simulink model "sampleModel2009"  (R2023a)
settings: Solver=VariableStepAuto  StartTime=0.0  StopTime=10.0  RelTol=1e-3
libraries: hdlsllib x4, simulink x3
settings Model: Creator=user1  LastModifiedBy=user1

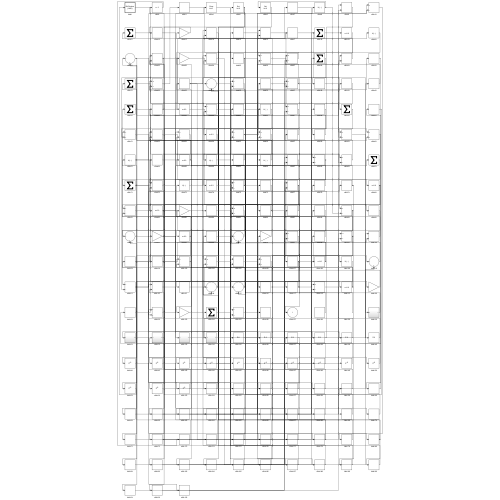
[thumbnail: Simulink's stored preview of the top-level diagram]
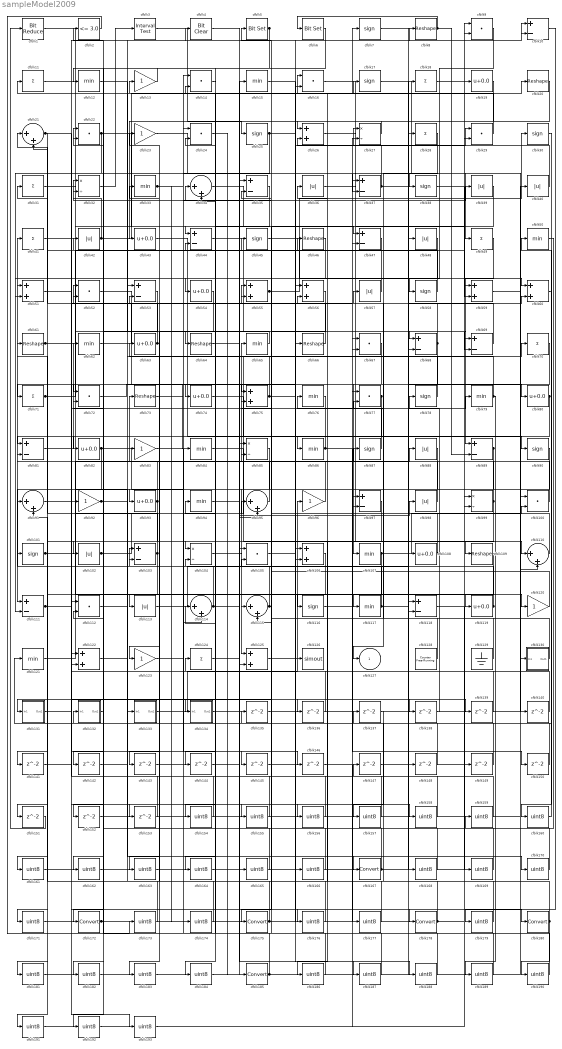
== system sampleModel2009 ==
  cfblk1 : hdlsllib/Logic and Bit Operations/Bit Reduce  mode=AND
  cfblk{10,35,37,44,47,53,68..69,81,89,97,103,111,118} (14 alike) : Sum  Inputs=+-
  cfblk{9,14,16,22,24,29,52,67,72,77,100,105,112} (13 alike) : DotProduct  OutDataTypeStr=Inherit: Inherit via internal rule
  cfblk{7,17,25,30,38,45,58,78,87,90,101,116} (12 alike) : Signum
  cfblk{36,39..40,42,48,57,88,98,102,113} (10 alike) : Abs  SaturateOnIntegerOverflow=off
  cfblk{27,32,85,99,104} (5 alike) : Product  Inputs=*/  RndMeth=Zero  SaturateOnIntegerOverflow=on
  cfblk{26,51,55..56,59..60,75,106,122,125} (10 alike) : Sum
  cfblk{12,15,33,50,62,65,76,79,84,86,94,107,117,121} (14 alike) : MinMax
  cfblk{19,43,54,63,74,80,82,93,108,119} (10 alike) : Bias  Bias=0.0  SaturateOnIntegerOverflow=off
  cfblk{8,20,46,61,64,66,73,109} (8 alike) : Reshape
  cfblk{11,18,28,31,41,49,70..71,124} (9 alike) : Sum  Inputs=+
  cfblk{21,34,91,95,110,114..115} (7 alike) : Sum  Inputs=|++
  cfblk{13,23,83,92,96,120,123} (7 alike) : Gain
  cfblk126 : ToWorkspace  VariableName=simout  SaveFormat=Timeseries  SampleTime=-1
  cfblk128 : hdlsllib/Sources/Counter Free-Running  NumBits=16  tsamp=-1
  cfblk129 : Ground
  cfblk130 : Subsystem
      settings: LibrarySourceBlock=|
      | hdlsllib/Ports &
      | Subsystems/Subsystem
  cfblk131 : Subsystem
      settings: LibrarySourceBlock=|
      | hdlsllib/Ports &
      | Subsystems/Subsystem
  cfblk132 : Subsystem
      settings: LibrarySourceBlock=|
      | hdlsllib/Ports &
      | Subsystems/Subsystem
  cfblk133 : Subsystem
      settings: LibrarySourceBlock=|
      | hdlsllib/Ports &
      | Subsystems/Subsystem
  cfblk134 : Subsystem
      settings: LibrarySourceBlock=|
      | hdlsllib/Ports &
      | Subsystems/Subsystem
  cfblk{135..153} (19 alike) : Delay  SampleTime=1
  cfblk{154..166,168..171,173..174,176..177,179,181..184,186..193} (34 alike) : DataTypeConversion  OutDataTypeStr=uint8  SaturateOnIntegerOverflow=off  RndMeth=Floor
  cfblk{167,172,175,178,180,185} (6 alike) : DataTypeConversion  SaturateOnIntegerOverflow=off  RndMeth=Floor
  cfblk2 : hdlsllib/Logic and Bit Operations/Compare To Constant  relop=<=  const=3.0  OutDataTypeStr=boolean
  cfblk3 : hdlsllib/Logic and Bit Operations/Interval Test  IntervalClosedRight=on  uplimit=0.5  IntervalClosedLeft=on  lowlimit=-0.5  OutDataTypeStr=boolean
  cfblk4 : simulink/Logic and Bit Operations/Bit Clear  iBit=0
      settings: LibrarySourceBlock=|
      | hdlsllib/Logic and Bit
      | Operations/Bit Clear
  cfblk5 : simulink/Logic and Bit Operations/Bit Set  iBit=0
      settings: LibrarySourceBlock=|
      | hdlsllib/Logic and Bit
      | Operations/Bit Set
  cfblk6 : simulink/Logic and Bit Operations/Bit Set  iBit=0
      settings: LibrarySourceBlock=|
      | hdlsllib/Logic and Bit
      | Operations/Bit Set
  cfblk127 : Outport  VectorParamsAs1DForOutWhenUnconnected=off
  wires:
  cfblk68/1 -> cfblk107/1, cfblk22/1, cfblk75/1
  cfblk11/1 -> cfblk44/1
  cfblk115/1 -> cfblk41/1, cfblk75/2
  cfblk20/1 -> cfblk104/1
  cfblk32/1 -> cfblk3/1
  cfblk75/1 -> cfblk131/1(In1), cfblk10/2, cfblk33/1
  cfblk16/1 -> cfblk38/1
  cfblk121/1 -> cfblk88/1
  cfblk17/1 -> cfblk49/1
  cfblk134/1(Out1) -> cfblk78/1
  cfblk41/1 -> cfblk119/1
  cfblk43/1 -> cfblk86/1
  cfblk45/1 -> cfblk60/1
  cfblk124/1 -> cfblk178/1
  cfblk66/1 -> cfblk21/1
  cfblk3/1 -> cfblk25/1
  cfblk86/1 -> cfblk81/1, cfblk139/1
  cfblk89/1 -> cfblk93/1, cfblk163/1
  cfblk8/1 -> cfblk6/1, cfblk89/2
  cfblk104/1 -> cfblk125/1
  cfblk128/1 -> cfblk13/1
  cfblk78/1 -> cfblk34/1
  cfblk95/1 -> cfblk51/1
  cfblk88/1 -> cfblk127/1
  cfblk25/1 -> cfblk111/2, cfblk144/1, cfblk158/1
  cfblk1/1 -> cfblk68/1
  cfblk36/1 -> cfblk110/1
  cfblk58/1 -> cfblk21/2
  cfblk111/1 -> cfblk92/1, cfblk79/1
  cfblk23/1 -> cfblk130/1(In1)
  cfblk55/1 -> cfblk30/1, cfblk29/1
  cfblk13/1 -> cfblk12/1
  cfblk133/1(Out1) -> cfblk96/1
  cfblk98/1 -> cfblk65/1
  cfblk80/1 -> cfblk183/1, cfblk184/1
  cfblk29/1 -> cfblk11/1
  cfblk6/1 -> cfblk74/1
  cfblk90/1 -> cfblk111/1
  cfblk53/1 -> cfblk172/1
  cfblk85/1 -> cfblk115/1
  cfblk93/1 -> cfblk81/2, cfblk181/1
  cfblk69/1 -> cfblk31/1
  cfblk5/1 -> cfblk134/1(In1), cfblk162/1
  cfblk34/1 -> cfblk47/1
  cfblk77/1 -> cfblk141/1, cfblk142/1
  cfblk84/1 -> cfblk109/1
  cfblk96/1 -> cfblk73/1
  cfblk64/1 -> cfblk20/1
  cfblk49/1 -> cfblk89/1
  cfblk60/1 -> cfblk121/1
  cfblk102/1 -> cfblk28/1, cfblk70/1
  cfblk26/1 -> cfblk59/1
  cfblk100/1 -> cfblk76/1
  cfblk9/1 -> cfblk58/1
  cfblk114/1 -> cfblk98/1, cfblk83/1
  cfblk72/1 -> cfblk84/1
  cfblk39/1 -> cfblk115/2
  cfblk37/1 -> cfblk27/1, cfblk80/1
  cfblk44/1 -> cfblk69/1
  cfblk103/1 -> cfblk113/1, cfblk61/1
  cfblk108/1 -> cfblk77/2, cfblk63/1
  cfblk92/1 -> cfblk120/1, cfblk138/1
  cfblk24/1 -> cfblk185/1
  cfblk28/1 -> cfblk117/1
  cfblk18/1 -> cfblk9/1
  cfblk33/1 -> cfblk17/1, cfblk37/2, cfblk174/1
  cfblk130/1(Out1) -> cfblk87/1
  cfblk27/1 -> cfblk26/1
  cfblk94/1 -> cfblk167/1
  cfblk42/1 -> cfblk7/1, cfblk32/2
  cfblk21/1 -> cfblk151/1, cfblk155/1
  cfblk38/1 -> cfblk59/2
  cfblk109/1 -> cfblk122/2
  cfblk87/1 -> cfblk26/2
  cfblk47/1 -> cfblk51/2
  cfblk101/1 -> cfblk27/2, cfblk145/1
  cfblk82/1 -> cfblk91/1, cfblk2/1, cfblk114/2, cfblk8/1
  cfblk57/1 -> cfblk54/1
  cfblk65/1 -> cfblk64/1
  cfblk54/1 -> cfblk123/1
  cfblk113/1 -> cfblk18/1
  cfblk71/1 -> cfblk9/2, cfblk153/1
  cfblk119/1 -> cfblk104/2, cfblk57/1
  cfblk74/1 -> cfblk90/1
  cfblk52/1 -> cfblk126/1
  cfblk19/1 -> cfblk43/1
  cfblk63/1 -> cfblk52/1, cfblk143/1
  cfblk62/1 -> cfblk37/1
  cfblk15/1 -> cfblk180/1
  cfblk61/1 -> cfblk133/1(In1), cfblk55/2
  cfblk91/1 -> cfblk4/1
  cfblk125/1 -> cfblk10/1
  cfblk122/1 -> cfblk46/1
  cfblk99/1 -> cfblk52/2, cfblk116/1, cfblk186/1
  cfblk81/1 -> cfblk62/1
  cfblk107/1 -> cfblk100/2, cfblk103/2, cfblk171/1
  cfblk117/1 -> cfblk60/2, cfblk55/1
  cfblk123/1 -> cfblk95/1
  cfblk76/1 -> cfblk82/1
  cfblk46/1 -> cfblk102/1
  cfblk48/1 -> cfblk72/1
  cfblk56/1 -> cfblk175/1
  cfblk22/1 -> cfblk95/2, cfblk71/1
  cfblk73/1 -> cfblk39/1
  cfblk31/1 -> cfblk66/1
  cfblk110/1 -> cfblk32/1
  cfblk79/1 -> cfblk23/1, cfblk189/1
  cfblk40/1 -> cfblk16/1
  cfblk12/1 -> cfblk69/2
  cfblk120/1 -> cfblk45/1
  cfblk129/1 -> cfblk103/1
  cfblk51/1 -> cfblk136/1
  cfblk136/1 -> cfblk122/1
  cfblk138/1 -> cfblk110/2
  cfblk139/1 -> cfblk44/2
  cfblk59/1 -> cfblk140/1
  cfblk140/1 -> cfblk99/1
  cfblk143/1 -> cfblk125/2
  cfblk145/1 -> cfblk29/2
  cfblk83/1 -> cfblk146/1
  cfblk147/1 -> cfblk68/2
  cfblk148/1 -> cfblk72/2
  cfblk149/1 -> cfblk85/2
  cfblk116/1 -> cfblk150/1
  cfblk150/1 -> cfblk91/2
  cfblk151/1 -> cfblk1/1
  cfblk70/1 -> cfblk152/1
  cfblk152/1 -> cfblk100/1
  cfblk153/1 -> cfblk22/2
  cfblk14/1 -> cfblk154/1
  cfblk154/1 -> cfblk112/2
  cfblk155/1 -> cfblk14/1
  cfblk142/1 -> cfblk156/1
  cfblk156/1 -> cfblk14/2
  cfblk137/1 -> cfblk157/1
  cfblk157/1 -> cfblk112/1
  cfblk158/1 -> cfblk137/1
  cfblk50/1 -> cfblk159/1
  cfblk159/1 -> cfblk135/1
  cfblk30/1 -> cfblk160/1
  cfblk160/1 -> cfblk50/1
  cfblk106/1 -> cfblk161/1
  cfblk161/1 -> cfblk148/1
  cfblk162/1 -> cfblk106/1
  cfblk163/1 -> cfblk106/2
  cfblk35/1 -> cfblk164/1
  cfblk164/1 -> cfblk48/1
  cfblk4/1 -> cfblk165/1
  cfblk165/1 -> cfblk35/1
  cfblk135/1 -> cfblk166/1
  cfblk166/1 -> cfblk35/2
  cfblk167/1 -> cfblk5/1, cfblk99/2
  cfblk7/1 -> cfblk168/1
  cfblk168/1 -> cfblk94/1
  cfblk118/1 -> cfblk169/1
  cfblk169/1 -> cfblk42/1
  cfblk112/1 -> cfblk170/1
  cfblk170/1 -> cfblk118/1
  cfblk171/1 -> cfblk118/2
  cfblk172/1 -> cfblk149/1, cfblk77/1
  cfblk2/1 -> cfblk173/1
  cfblk173/1 -> cfblk53/1
  cfblk174/1 -> cfblk53/2
  cfblk175/1 -> cfblk16/2, cfblk114/1
  cfblk131/1(Out1) -> cfblk176/1
  cfblk176/1 -> cfblk56/1
  cfblk146/1 -> cfblk177/1
  cfblk177/1 -> cfblk56/2
  cfblk178/1 -> cfblk101/1, cfblk36/1
  cfblk10/1 -> cfblk179/1
  cfblk179/1 -> cfblk124/1
  cfblk180/1 -> cfblk147/1, cfblk34/2, cfblk190/1
  cfblk181/1 -> cfblk15/1
  cfblk97/1 -> cfblk182/1
  cfblk182/1 -> cfblk108/1
  cfblk183/1 -> cfblk97/1
  cfblk184/1 -> cfblk97/2
  cfblk185/1 -> cfblk40/1, cfblk85/1, cfblk47/2
  cfblk186/1 -> cfblk24/1
  cfblk144/1 -> cfblk187/1
  cfblk187/1 -> cfblk24/2
  cfblk105/1 -> cfblk188/1
  cfblk188/1 -> cfblk132/1(In1)
  cfblk189/1 -> cfblk105/1
  cfblk190/1 -> cfblk105/2
  cfblk67/1 -> cfblk191/1
  cfblk191/1 -> cfblk19/1
  cfblk132/1(Out1) -> cfblk192/1
  cfblk192/1 -> cfblk67/1
  cfblk141/1 -> cfblk193/1
  cfblk193/1 -> cfblk67/2

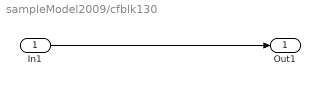
== system sampleModel2009/cfblk130 ==
  In1 : Inport
  Out1 : Outport
  wires:
  In1/1 -> Out1/1

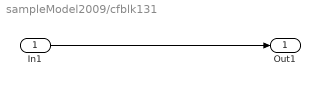
== system sampleModel2009/cfblk131 ==
  In1 : Inport
  Out1 : Outport
  wires:
  In1/1 -> Out1/1

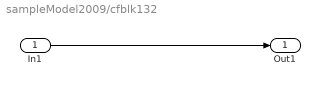
== system sampleModel2009/cfblk132 ==
  In1 : Inport
  Out1 : Outport
  wires:
  In1/1 -> Out1/1

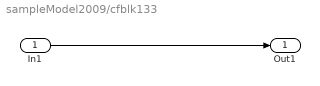
== system sampleModel2009/cfblk133 ==
  In1 : Inport
  Out1 : Outport
  wires:
  In1/1 -> Out1/1

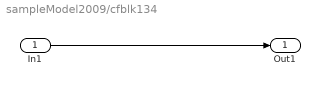
== system sampleModel2009/cfblk134 ==
  In1 : Inport
  Out1 : Outport
  wires:
  In1/1 -> Out1/1
